simulink model "longDriverSimple"  (R2018a)
settings: Solver=VariableStepAuto  StartTime=0.0  StopTime=10.0  RelTol=1e-3
undefined symbols (not defined in the file): ctl
libraries: autolibshared x1
settings Model: Creator=carca  LastModifiedBy=carca

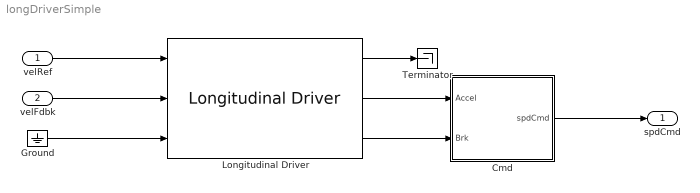
== system longDriverSimple ==
  velRef : Inport
  velFdbk : Inport  Port=2
  Cmd : Subsystem
  Ground : Ground
  Longitudinal Driver : autolibshared/Longitudinal Driver  aMode=1  vnom=100  Kp=ctl.Kp  Ki=ctl.Ki  Kaw=.1  Kff=ctl.kff  Kg=.01  tauerr=.03
      settings: SourceProductName=Powertrain Blockset  SourceProductBaseCode=PW
  Terminator : Terminator
  spdCmd : Outport
  wires:
  Ground/1 -> Longitudinal Driver/3
  velFdbk/1 -> Longitudinal Driver/2
  velRef/1 -> Longitudinal Driver/1
  Longitudinal Driver/2 -> Cmd/1(Accel)
  Longitudinal Driver/3 -> Cmd/2(Brk)
  Cmd/1(spdCmd) -> spdCmd/1
  Longitudinal Driver/1 -> Terminator/1

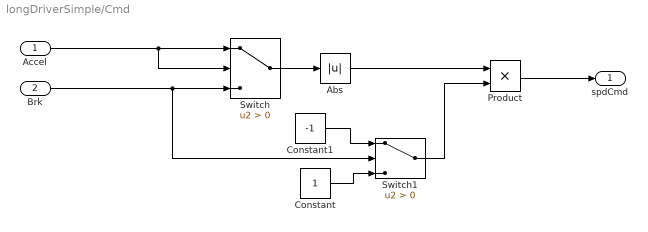
== system longDriverSimple/Cmd ==
  Accel : Inport
  Brk : Inport  Port=2
  Abs : Abs
  Constant : Constant
  Constant1 : Constant  Value=-1
  Product : Product
  Switch : Switch  Criteria=u2 > Threshold
  Switch1 : Switch  Criteria=u2 > Threshold
  spdCmd : Outport
  wires:
  Switch/1 -> Abs/1
  Accel/1 -> Switch/2, Switch/1
  Constant1/1 -> Switch1/1
  Abs/1 -> Product/1
  Switch1/1 -> Product/2
  Constant/1 -> Switch1/3
  Brk/1 -> Switch1/2, Switch/3
  Product/1 -> spdCmd/1
